simulink model "mimo"  (Simulink 6.6)
settings: Solver=ode45  StartTime=0.0  StopTime=10.0  RelTol=1e-3
libraries: dspindex x18, commchan2 x16, commchan3 x4, commdigbbndpm2 x3, commrandsrc2 x1, dspsrcs4 x1, commsink2 x1, dspobslib x1, dspinverses x1, dspmtrx3 x1
settings Model: Creator=a  LastModifiedBy=a

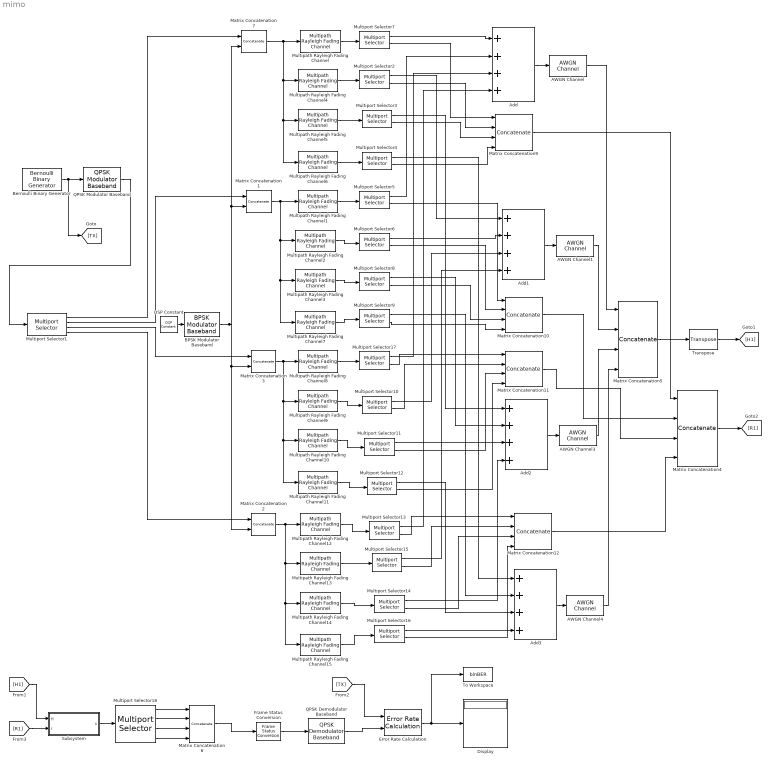
== system mimo ==
  AWGN Channel : commchan3/AWGN Channel  SystemSampleTime=-1  seed=67  noiseMode="Signal to noise ratio  (SNR)"  EbNodB=20  EsNodB=10  SNRdB=0  bitsPerSym=1  Ps=1  Tsym=1e-3/3  variance=1
  AWGN Channel1 : commchan3/AWGN Channel  SystemSampleTime=-1  seed=68  noiseMode="Signal to noise ratio  (SNR)"  EbNodB=20  EsNodB=10  SNRdB=0  bitsPerSym=1  Ps=1  Tsym=1e-3/3  variance=1
  AWGN Channel3 : commchan3/AWGN Channel  SystemSampleTime=-1  seed=69  noiseMode="Signal to noise ratio  (SNR)"  EbNodB=20  EsNodB=10  SNRdB=0  bitsPerSym=1  Ps=1  Tsym=1e-3/3  variance=1
  AWGN Channel4 : commchan3/AWGN Channel  SystemSampleTime=-1  seed=70  noiseMode="Signal to noise ratio  (SNR)"  EbNodB=20  EsNodB=10  SNRdB=0  bitsPerSym=1  Ps=1  Tsym=1e-3/3  variance=1
  Add{,1..3} (4 alike) : Sum  Inputs=4  OutScaling=2^-10
  BPSK Modulator Baseband : commdigbbndpm2/BPSK Modulator Baseband  SystemSampleTime=-1  Ph=0  numSamp=1
  Bernoulli Binary Generator : commrandsrc2/Bernoulli Binary Generator  DialogController=commDDGCreate  DialogControllerArgs=DataTag0  SystemSampleTime=-1  P=0.5  seed=61  Ts=1e-6/16/2  frameBased=on  sampPerFrame=32  orient=off  outDataType=double
  DSP Constant : dspsrcs4/DSP Constant  SystemSampleTime=-1  Value=0  SampleMode=Discrete  discreteOutput=Frame-based  continuousOutput=Sample-based  sampTime=1e-3/64  framePeriod=1e-6  dataType=Inherit from 'Constant value'  isSigned=on  wordLen=16  udDataType=sfix(16)  fracBitsMode=Best precision  numFracBits=15  InterpretAs1D=-inf  Ts=-inf  FramebasedOutput=-inf
  Display : Display
  Error Rate Calculation : commsink2/Error Rate Calculation  N=0  st_delay=0  cp_mode=Entire frame  subframe=[]  PMode=Port  WsName=ErrorVec  RsMode2=off  stop=on  numErr=1e6  maxBits=1e6
  Frame Status Conversion : dspobslib/Frame Status Conversion  SystemSampleTime=-1  growRefPort=off  outframe=Frame-based
  Matrix Concatenation{1..3,7} (4 alike) : Concatenate  Mode=Multidimensional array
  Matrix Concatenation{6,9..12} (5 alike) : Concatenate  NumInputs=4  Mode=Multidimensional array
  Matrix Concatenation4 : Concatenate  NumInputs=4  Mode=Multidimensional array  ConcatenateDimension=2
  Matrix Concatenation5 : Concatenate  NumInputs=4  Mode=Multidimensional array  ConcatenateDimension=2
  Multipath Rayleigh Fading Channel : commchan2/Multipath Rayleigh Fading Channel  SystemSampleTime=-1  Fd=100  simTs=1e-6/5  delayVec=[0]  gainVecdB=[0]  normGain=on  Seed=71
  Multipath Rayleigh Fading Channel1 : commchan2/Multipath Rayleigh Fading Channel  SystemSampleTime=-1  Fd=100  simTs=1e-6/5  delayVec=[0]  gainVecdB=[0]  normGain=on  Seed=75
  Multipath Rayleigh Fading Channel10 : commchan2/Multipath Rayleigh Fading Channel  SystemSampleTime=-1  Fd=100  simTs=1e-6/5  delayVec=[0]  gainVecdB=[0]  normGain=on  Seed=81
  Multipath Rayleigh Fading Channel11 : commchan2/Multipath Rayleigh Fading Channel  SystemSampleTime=-1  Fd=100  simTs=1e-6/5  delayVec=[0]  gainVecdB=[0]  normGain=on  Seed=82
  Multipath Rayleigh Fading Channel12 : commchan2/Multipath Rayleigh Fading Channel  SystemSampleTime=-1  Fd=100  simTs=1e-6/5  delayVec=[0]  gainVecdB=[0]  normGain=on  Seed=83
  Multipath Rayleigh Fading Channel13 : commchan2/Multipath Rayleigh Fading Channel  SystemSampleTime=-1  Fd=100  simTs=1e-6/5  delayVec=[0]  gainVecdB=[0]  normGain=on  Seed=84
  Multipath Rayleigh Fading Channel14 : commchan2/Multipath Rayleigh Fading Channel  SystemSampleTime=-1  Fd=100  simTs=1e-6/5  delayVec=[0]  gainVecdB=[0]  normGain=on  Seed=85
  Multipath Rayleigh Fading Channel15 : commchan2/Multipath Rayleigh Fading Channel  SystemSampleTime=-1  Fd=100  simTs=1e-6/5  delayVec=[0]  gainVecdB=[0]  normGain=on  Seed=86
  Multipath Rayleigh Fading Channel2 : commchan2/Multipath Rayleigh Fading Channel  SystemSampleTime=-1  Fd=100  simTs=1e-6/5  delayVec=[0]  gainVecdB=[0]  normGain=on  Seed=76
  Multipath Rayleigh Fading Channel3 : commchan2/Multipath Rayleigh Fading Channel  SystemSampleTime=-1  Fd=100  simTs=1e-6/5  delayVec=[0]  gainVecdB=[0]  normGain=on  Seed=77
  Multipath Rayleigh Fading Channel4 : commchan2/Multipath Rayleigh Fading Channel  SystemSampleTime=-1  Fd=100  simTs=1e-6/5  delayVec=[0]  gainVecdB=[0]  normGain=on  Seed=72
  Multipath Rayleigh Fading Channel5 : commchan2/Multipath Rayleigh Fading Channel  SystemSampleTime=-1  Fd=100  simTs=1e-6/5  delayVec=[0 ]  gainVecdB=[0 ]  normGain=on  Seed=73
  Multipath Rayleigh Fading Channel6 : commchan2/Multipath Rayleigh Fading Channel  SystemSampleTime=-1  Fd=100  simTs=1e-6/5  delayVec=[0 ]  gainVecdB=[0 ]  normGain=on  Seed=74
  Multipath Rayleigh Fading Channel7 : commchan2/Multipath Rayleigh Fading Channel  SystemSampleTime=-1  Fd=100  simTs=1e-6/5  delayVec=[0]  gainVecdB=[0]  normGain=on  Seed=78
  Multipath Rayleigh Fading Channel8 : commchan2/Multipath Rayleigh Fading Channel  SystemSampleTime=-1  Fd=100  simTs=1e-6/5  delayVec=[0]  gainVecdB=[0]  normGain=on  Seed=79
  Multipath Rayleigh Fading Channel9 : commchan2/Multipath Rayleigh Fading Channel  SystemSampleTime=-1  Fd=100  simTs=1e-6/5  delayVec=[0]  gainVecdB=[0]  normGain=on  Seed=80
  Multiport Selector1 : dspindex/Multiport Selector  rowsOrCols=Rows  idxCellArray={ [1 5 9 13],[2 6 10 14],[3 7 11 15],[4 8 12 16] }  idxErrMode=Clip Index
  Multiport Selector{2..17} (16 alike) : dspindex/Multiport Selector  rowsOrCols=Rows  idxCellArray={ [1:1:4],5 }  idxErrMode=Clip Index
  Multiport Selector18 : dspindex/Multiport Selector  rowsOrCols=Columns  idxCellArray={ [1],[2],[3],[4] }  idxErrMode=Clip Index
  QPSK Demodulator Baseband : commdigbbndpm2/QPSK Demodulator Baseband  SystemSampleTime=-1  OutType=Bit  Dec=Binary  Ph=pi/4  numSamp=1
  QPSK Modulator Baseband : commdigbbndpm2/QPSK Modulator Baseband  SystemSampleTime=-1  InType=Bit  Enc=Binary  Ph=pi/4  numSamp=1
  Subsystem : Subsystem
  To Workspace : ToWorkspace  VariableName=binBER  SampleTime=-1  SaveFormat=Array
      settings: MaxDataPoints=1
  Transpose : dspmtrx3/Transpose  SystemSampleTime=-1  Hermitian=off  overflowFlag=off
  wires:
  Matrix Concatenation7/1 -> Multipath Rayleigh Fading Channel/1, Multipath Rayleigh Fading Channel4/1, Multipath Rayleigh Fading Channel5/1, Multipath Rayleigh Fading Channel6/1
  Matrix Concatenation1/1 -> Multipath Rayleigh Fading Channel7/1, Multipath Rayleigh Fading Channel3/1, Multipath Rayleigh Fading Channel2/1, Multipath Rayleigh Fading Channel1/1
  Multipath Rayleigh Fading Channel/1 -> Multiport Selector7/1
  Multipath Rayleigh Fading Channel4/1 -> Multiport Selector2/1
  Multipath Rayleigh Fading Channel5/1 -> Multiport Selector3/1
  Multipath Rayleigh Fading Channel6/1 -> Multiport Selector4/1
  Multipath Rayleigh Fading Channel1/1 -> Multiport Selector5/1
  Multipath Rayleigh Fading Channel2/1 -> Multiport Selector6/1
  Multipath Rayleigh Fading Channel3/1 -> Multiport Selector8/1
  Multipath Rayleigh Fading Channel7/1 -> Multiport Selector9/1
  Matrix Concatenation3/1 -> Multipath Rayleigh Fading Channel10/1, Multipath Rayleigh Fading Channel11/1, Multipath Rayleigh Fading Channel9/1, Multipath Rayleigh Fading Channel8/1
  Matrix Concatenation2/1 -> Multipath Rayleigh Fading Channel14/1, Multipath Rayleigh Fading Channel15/1, Multipath Rayleigh Fading Channel13/1, Multipath Rayleigh Fading Channel12/1
  Multipath Rayleigh Fading Channel8/1 -> Multiport Selector17/1
  Multipath Rayleigh Fading Channel9/1 -> Multiport Selector10/1
  Multipath Rayleigh Fading Channel10/1 -> Multiport Selector11/1
  Multipath Rayleigh Fading Channel11/1 -> Multiport Selector12/1
  Multipath Rayleigh Fading Channel12/1 -> Multiport Selector13/1
  Multipath Rayleigh Fading Channel14/1 -> Multiport Selector14/1
  Multipath Rayleigh Fading Channel15/1 -> Multiport Selector16/1
  Multipath Rayleigh Fading Channel13/1 -> Multiport Selector15/1
  DSP Constant/1 -> BPSK Modulator Baseband/1
  BPSK Modulator Baseband/1 -> Matrix Concatenation7/2, Matrix Concatenation1/2, Matrix Concatenation2/2, Matrix Concatenation3/2
  Multiport Selector7/1 -> Add/1
  Multiport Selector5/1 -> Add/2
  Multiport Selector17/1 -> Add/3
  Multiport Selector13/1 -> Add/4
  Multiport Selector2/1 -> Add1/1
  Multiport Selector6/1 -> Add1/2
  Multiport Selector10/1 -> Add1/3
  Multiport Selector15/1 -> Add1/4
  Multiport Selector3/1 -> Add2/1
  Multiport Selector8/1 -> Add2/2
  Multiport Selector11/1 -> Add2/3
  Multiport Selector14/1 -> Add2/4
  Multiport Selector4/1 -> Add3/1
  Multiport Selector9/1 -> Add3/2
  Multiport Selector12/1 -> Add3/3
  Multiport Selector16/1 -> Add3/4
  Multiport Selector7/2 -> Matrix Concatenation9/1
  Multiport Selector2/2 -> Matrix Concatenation9/2
  Multiport Selector3/2 -> Matrix Concatenation9/3
  Multiport Selector4/2 -> Matrix Concatenation9/4
  Multiport Selector5/2 -> Matrix Concatenation10/1
  Multiport Selector6/2 -> Matrix Concatenation10/2
  Multiport Selector8/2 -> Matrix Concatenation10/3
  Multiport Selector9/2 -> Matrix Concatenation10/4
  Multiport Selector17/2 -> Matrix Concatenation11/1
  Multiport Selector10/2 -> Matrix Concatenation11/2
  Multiport Selector11/2 -> Matrix Concatenation11/3
  Multiport Selector12/2 -> Matrix Concatenation11/4
  Multiport Selector13/2 -> Matrix Concatenation12/1
  Multiport Selector15/2 -> Matrix Concatenation12/2
  Multiport Selector14/2 -> Matrix Concatenation12/3
  Multiport Selector16/2 -> Matrix Concatenation12/4
  Add/1 -> AWGN Channel/1
  Add1/1 -> AWGN Channel1/1
  Add2/1 -> AWGN Channel3/1
  Add3/1 -> AWGN Channel4/1
  AWGN Channel/1 -> Matrix Concatenation5/1
  AWGN Channel1/1 -> Matrix Concatenation5/2
  AWGN Channel3/1 -> Matrix Concatenation5/3
  AWGN Channel4/1 -> Matrix Concatenation5/4
  Matrix Concatenation5/1 -> Transpose/1
  Matrix Concatenation9/1 -> Matrix Concatenation4/1
  Matrix Concatenation10/1 -> Matrix Concatenation4/2
  Matrix Concatenation11/1 -> Matrix Concatenation4/3
  Matrix Concatenation12/1 -> Matrix Concatenation4/4
  Subsystem/1(x) -> Multiport Selector18/1
  Multiport Selector18/1 -> Matrix Concatenation6/1
  Multiport Selector18/2 -> Matrix Concatenation6/2
  Multiport Selector18/3 -> Matrix Concatenation6/3
  Multiport Selector18/4 -> Matrix Concatenation6/4
  Bernoulli Binary Generator/1 -> QPSK Modulator Baseband/1, [TX]
  QPSK Modulator Baseband/1 -> Multiport Selector1/1
  Multiport Selector1/1 -> Matrix Concatenation7/1
  Multiport Selector1/2 -> Matrix Concatenation1/1
  Multiport Selector1/3 -> Matrix Concatenation3/1
  Multiport Selector1/4 -> Matrix Concatenation2/1
  Matrix Concatenation6/1 -> Frame Status Conversion/1
  Frame Status Conversion/1 -> QPSK Demodulator Baseband/1
  QPSK Demodulator Baseband/1 -> Error Rate Calculation/2
  Error Rate Calculation/1 -> Display/1, To Workspace/1
  [TX] -> Error Rate Calculation/1
  [H1] -> Subsystem/1(H)
  [R1] -> Subsystem/2(r)
  Transpose/1 -> [H1]
  Matrix Concatenation4/1 -> [R1]

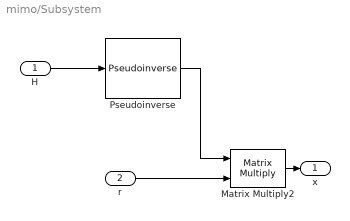
== system mimo/Subsystem ==
  H : Inport
  r : Inport  Port=2
  Matrix Multiply2 : Product  Multiplication=Matrix(*)
  Pseudoinverse : dspinverses/Pseudoinverse  wanterr=off
  x : Outport
  wires:
  H/1 -> Pseudoinverse/1
  r/1 -> Matrix Multiply2/2
  Matrix Multiply2/1 -> x/1
  Pseudoinverse/1 -> Matrix Multiply2/1
